simulink model "Falcon_simulink"  (R2019a)
settings: Solver=VariableStepAuto  StartTime=0.0  StopTime=2.5  RelTol=1e-3
undefined symbols (not defined in the file): A1, A2, C_d1, C_d2, g, m, rho
settings Model: Creator=aleri934  LastModifiedBy=aleri934

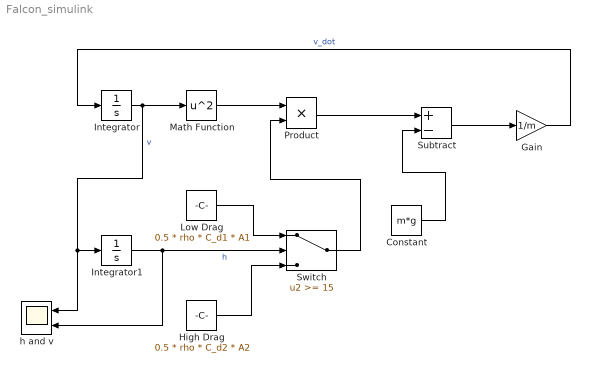
== system Falcon_simulink ==
  Constant : Constant  Value=m*g
  Gain : Gain  Gain=1/m
  High Drag : Constant  Value=0.5 * rho * C_d2 * A2
  Integrator : Integrator  InitialCondition=-10
  Integrator1 : Integrator  InitialCondition=60
  Low Drag : Constant  Value=0.5 * rho * C_d1 * A1
  Math Function : Math  Operator=square  SaturateOnIntegerOverflow=on
  Product : Product
  Subtract : Sum  Inputs=+-
  Switch : Switch  Threshold=15
  h and v : Scope  NumInputPorts=2
  wires:
  Integrator/1 -> h and v/1, Integrator1/1, Math Function/1  "v"
  Gain/1 -> Integrator/1  "v_dot"
  Low Drag/1 -> Switch/1
  High Drag/1 -> Switch/3
  Math Function/1 -> Product/1
  Switch/1 -> Product/2
  Constant/1 -> Subtract/2
  Product/1 -> Subtract/1
  Subtract/1 -> Gain/1
  Integrator1/1 -> h and v/2, Switch/2  "h"
